simulink model "amesimcar_pathplannerv2"  (R2018b)
settings: Solver=VariableStepAuto  StartTime=0.0  StopTime=Tf  RelTol=1e-3
values from neighbouring files (symbols this model uses):
  centerline1 = line_data.centerline_right    [main.m]
  left_line = line_data.left_line    [main.m]
  right_line = line_data.right_line    [main.m]
undefined symbols (not defined in the file or in its folder): PlanningFunction
libraries: simulink x1
settings Model: Creator=pm6kgn  LastModifiedBy=t2vosx
settings DebuggingCC: LibraryContextMissingDiagnostic=none
settings SFSimCC: SimUseLocalCustomCode=off
settings RTWCC: RTWUseLocalCustomCode=off

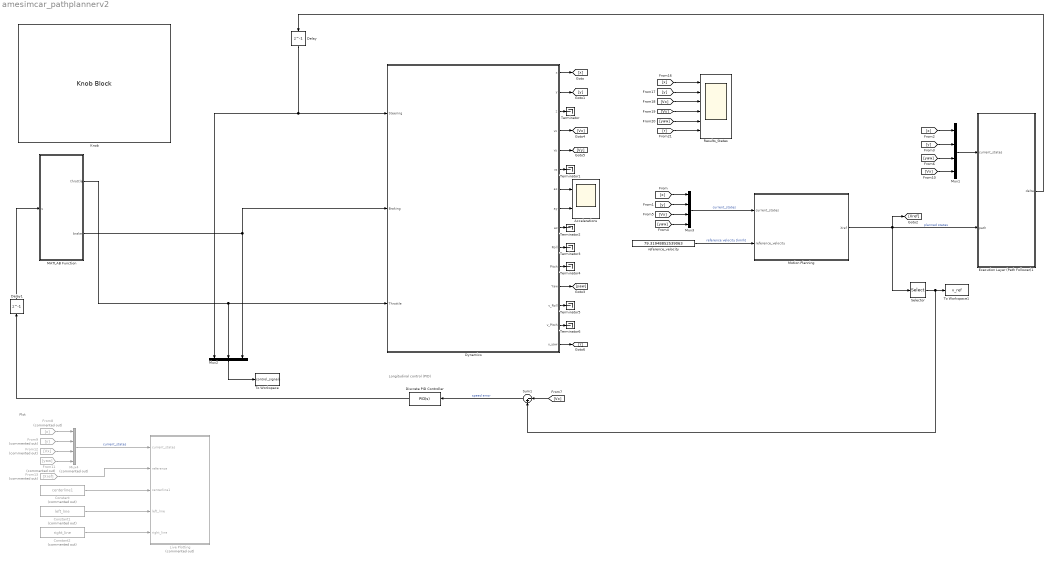
== system amesimcar_pathplannerv2 ==
  note: Plot
  note: Longitudinal control (PID)
  Accelerations : Scope  NumInputPorts=2
  Constant : Constant  Commented=on  Value=centerline1
  Constant1 : Constant  Commented=on  Value=left_line
  Constant2 : Constant  Commented=on  Value=right_line
  Delay : Delay  DelayLength=1  InitialCondition=0
  Delay1 : Delay  DelayLength=1  InitialCondition=0
  Discrete PID Controller : simulink/Continuous/PID Controller  Controller=PID  Form=Parallel  TimeDomain=Continuous-time  SampleTime=-1  IntegratorMethod=Forward Euler  FilterMethod=Forward Euler  ControllerParametersSource=internal  P=0.1  I=0.01  D=0  UseFilter=on  N=100  TunerSelectOption=Transfer Function Based (PID Tuner App)  InitialConditionSource=internal  InitialConditionForIntegrator=0  InitialConditionForFilter=0  DifferentiatorICPrevScaledInput=0  ExternalReset=none  TrackingMode=off  Kt=1  LimitOutput=on  UpperSaturationLimit=1  LowerSaturationLimit=-1  LinearizeAsGain=off  AntiWindupMode=none  Kb=1  POutMin=[]  POutMax=[]  IOutMin=[]  IOutMax=[]  DOutMin=[]  DOutMax=[]  NOutMin=[]  NOutMax=[]  SumOutMin=[]  SumOutMax=[]  SaturationOutMin=[]  SaturationOutMax=[]  PParamMin=[]  PParamMax=[]  IParamMin=[]  IParamMax=[]  DParamMin=[]  DParamMax=[]  NParamMin=[]  NParamMax=[]  KbParamMin=[]  KbParamMax=[]  KtParamMin=[]  KtParamMax=[]  KbOutMin=[]  KbOutMax=[]  KtOutMin=[]  KtOutMax=[]  IntegratorOutMin=[]  IntegratorOutMax=[]  FilterOutMin=[]  FilterOutMax=[]  SumI1OutMin=[]  SumI1OutMax=[]  SumI2OutMin=[]  SumI2OutMax=[]  SumI3OutMin=[]  SumI3OutMax=[]  SumI4OutMin=[]  SumI4OutMax=[]  SumDOutMin=[]  SumDOutMax=[]  DifferentiatorOutMin=[]  DifferentiatorOutMax=[]  FilterDiffOutCoefMin=[]  FilterDiffOutCoefMax=[]  ReciprocalOutMin=[]  ReciprocalOutMax=[]  SumDenOutMin=[]  SumDenOutMax=[]  SumNumOutMin=[]  SumNumOutMax=[]  DivideOutMin=[]  DivideOutMax=[]  IntegratorContinuousStateAttributes=''  IntegratorStateMustResolveToSignalObject=off  IntegratorRTWStateStorageClass=Auto  FilterContinuousStateAttributes=''  FilterStateMustResolveToSignalObject=off  FilterRTWStateStorageClass=Auto  ParallelPVariant=InternalParameters  IdealPVariant=Disabled  IVariant=InternalParameters  DVariant=InternalParameters  IntegratorVariant=Continuous  SatVariant=Enabled  AWVariant=Passthrough  PCopyVariant=Disabled  TRVariant=Disabled  FdbkBlocksVariant=Forward  IdealPFdbkVariant=Disabled  SatFdbkVariant=Disabled  DerivativeFilterVariant=ContFilter  NVariant=InternalParameters  NCopyVariant=Disabled  FilterICVariant=InternalICsFilter  IntegratorICVariant=InternalICs  ExternalResetVariant=Disabled  TRSumVariant=Passthrough  SumFdbkVariant=Disabled  SumVariant=Sum_PID
  Dynamics : Subsystem  Tag=AME2SLCoSim  InitFcn=AMESimLib_initBlock  StartFcn=AMESimLib_startBlock  StopFcn=AMESimLib_stopBlock
      settings: DeleteFcn=AMESimLib_deleteBlock  OpenFcn=AMESimLib_openBlock('AME2SLCoSim')
      mask Display: image(imread('amesim_pix256.png'),[0.4,0.7,0.2,0.2]);disp('Simcenter Amesim co-Sim:\nDynamics');port_label('input',1,'Steering');port_label('input',2,'Braking');port_label('input',3,'Throttle');port_label('output',1,'x');port_label('output',2,'y');port_label('output',3,'z');port_label('output',4,'vx');port_label('output',5,'vy');port_label('output',6,'vz');port_label('output',7,'ax');port_label('output',8,'ay');port_label('output',9,'az');port_label('output',10,'Roll');port_label('output',11,'Pitch');port_label('output',12,'Yaw');port_label('output',13,'v_Roll');port_label('output',14,'v_Pitch');port_label('output',15,'v_yaw');
  Execution Layer (Path Follower)1 : MATLAB Function  TreatAsAtomicUnit=on  SystemSampleTime=0.01
  From11 : From  Commented=on  GotoTag=yaw
  From12 : From  Commented=on  GotoTag=Vx
  From13 : From  Commented=on  GotoTag=Xref
  From8 : From  Commented=on  GotoTag=x
  From9 : From  Commented=on  GotoTag=y
  Knob : KnobBlock  WebBlockId=204  ScaleMin=5  ScaleMax=80
  Live Plotting : MATLAB Function  Commented=on  TreatAsAtomicUnit=on
  MATLAB Function : MATLAB Function  TreatAsAtomicUnit=on
  Motion Planning : Subsystem  TreatAsAtomicUnit=on  SystemSampleTime=0.1
      mask Display: image('C:\Users\pm6kgn\Documents\Images\2479573.png');
  Mux1 : Mux
  Mux2 : Mux  Inputs=3
  Mux3 : Mux
  Mux4 : Mux  Commented=on
  Results_States : Scope  NumInputPorts=6
  Selector : Selector  NumberOfDimensions=2  InputPortWidth=[4 50]  IndexOptions=Index vector (dialog),Index vector (dialog)  Indices=3,50  OutputSizes=1,1
  Sum1 : Sum  Inputs=|-+
  Terminator{,1..6} (7 alike) : Terminator
  To Workspace : ToWorkspace  VariableName=control_signals  SaveFormat=Structure With Time  SampleTime=-1
  To Workspace1 : ToWorkspace  VariableName=v_ref  SaveFormat=Timeseries  SampleTime=-1
  reference_velocity : Constant  Value=79.31948852539063
  wires:
  MATLAB Function/1(throttle) -> Dynamics/3(Throttle), Mux2/2
  MATLAB Function/2(brake) -> Mux2/3, Dynamics/2(Braking)
  Mux2/1 -> To Workspace/1
  Sum1/1 -> Discrete PID Controller/1  "speed error"
  Mux1/1 -> Execution Layer (Path Follower)1/1(current_states)
  Dynamics/1(x) -> [x]
  Dynamics/4(vx) -> [Vx]
  Dynamics/2(y) -> [y]
  [x] -> Mux1/1
  [y] -> Mux1/2
  Dynamics/12(Yaw) -> [yaw]
  [yaw] -> Mux1/3
  Discrete PID Controller/1 -> Delay1/1
  [Vx] -> Sum1/1
  Delay1/1 -> MATLAB Function/1(u)
  Dynamics/7(ax) -> Accelerations/1
  Dynamics/8(ay) -> Accelerations/2
  Delay/1 -> Dynamics/1(Steering), Mux2/1
  [Vx] -> Mux1/4
  Execution Layer (Path Follower)1/1(delta) -> Delay/1
  Dynamics/5(vy) -> [Vy]
  Dynamics/15(v_yaw) -> [r]
  [x] -> Results_States/1
  [y] -> Results_States/2
  [Vx] -> Results_States/3
  [Vy] -> Results_States/4
  [r] -> Results_States/6
  [yaw] -> Results_States/5
  Selector/1 -> Sum1/2, To Workspace1/1
  Motion Planning/1(Xref) -> [Xref], Selector/1, Execution Layer (Path Follower)1/2(path)  "planned states"
  [y] -> Mux3/2
  [x] -> Mux3/1
  [yaw] -> Mux3/4
  Mux3/1 -> Motion Planning/1("current_states ")  "current_states"
  [Vx] -> Mux3/3
  reference_velocity/1 -> Motion Planning/2(reference_velocity)  "reference velocity [km/h]"
  Dynamics/3(z) -> Terminator/1
  Dynamics/6(vz) -> Terminator1/1
  Dynamics/9(az) -> Terminator2/1
  Dynamics/10(Roll) -> Terminator3/1
  Dynamics/11(Pitch) -> Terminator4/1
  Dynamics/13(v_Roll) -> Terminator5/1
  Dynamics/14(v_Pitch) -> Terminator6/1
  From8/1 -> Mux4/1
  From9/1 -> Mux4/2
  Mux4/1 -> Live Plotting/1(current_states)  "current_states"
  From12/1 -> Mux4/3
  From11/1 -> Mux4/4
  From13/1 -> Live Plotting/2(reference)
  Constant/1 -> Live Plotting/3(centerline1)
  Constant1/1 -> Live Plotting/4(left_line)
  Constant2/1 -> Live Plotting/5(right_line)

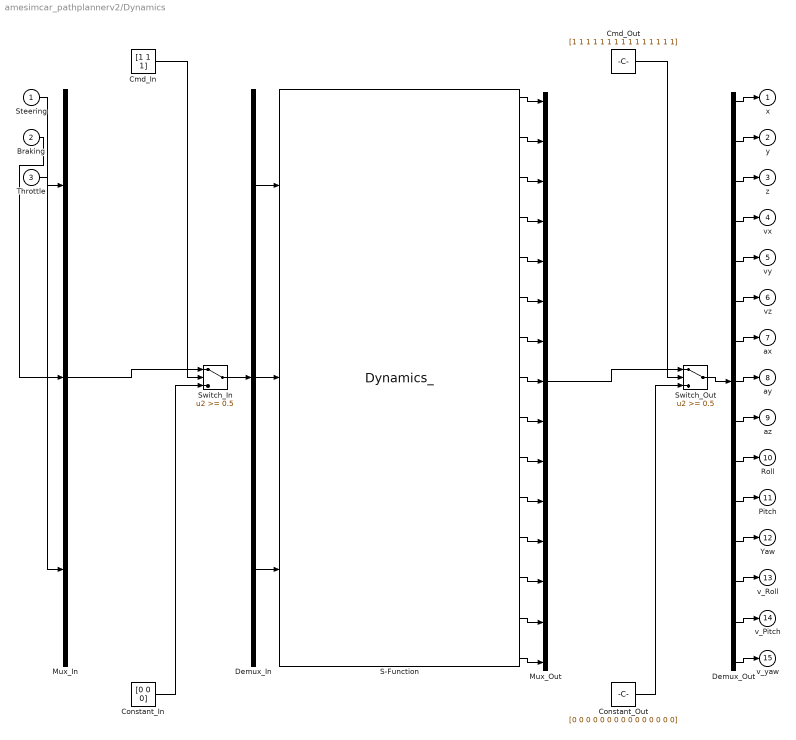
== system amesimcar_pathplannerv2/Dynamics ==
  Steering : Inport
  Braking : Inport  Port=2
  Throttle : Inport  Port=3
  Cmd_In : Constant  Value=[1 1 1]
  Cmd_Out : Constant  Value=[1 1 1 1 1 1 1 1 1 1 1 1 1 1 1]
  Constant_In : Constant  Value=[0 0 0]
  Constant_Out : Constant  Value=[0 0 0 0 0 0 0 0 0 0 0 0 0 0 0]
  Demux_In : Demux  Outputs=3
  Demux_Out : Demux  Outputs=15
  Mux_In : Mux  Inputs=3
  Mux_Out : Mux  Inputs=15
  S-Function : S-Function  InitFcn=clear Dynamics_  StopFcn=clear Dynamics_  FunctionName=Dynamics_  Parameters="[0.01;0.01;1e-05;1e+30;100;0;0;2;0;1;0.001;0;1] ['Grav           ';'Xg             ';'Zg             ';'V0             ';'Msprung        ';'Msteer         ';'Msp_front      ';'Mwh_front      ';'Msp_rear       ';'Mwh_rear       ';'Isprung_xx     ';'Isprung_yy     ';'Isprung_zz     ';'Isprung_xy     ';'Isprung_xz     ';'Isprung_yz     ';'Zref_front     ';'Zref_rear      ';'wheelbase      ';'track_front    ';'track_rear     ';'Rpinion        ';'Ksusp_front    ';'Ksusp_rear     ';'Rsusp_front    ';'Rsusp_rear     ';'Kantiroll_front';'Kantiroll_rear ';'Rfree          ';'Rroll          ';'Ktire          ';'Rtire          ';'a1             ';'a2             ';'a3             ';'a4             '] [9.8066;1056;375;0;1300;2;18;18;15;14;250;1000;1300;0;-20;0;75;75;2400;1450;1450;8;21000;21000;2000;1500;30000;20000;0.292;0.291;200000;100;-50;1200;1000;5] [] [] [] []"  SFunctionDeploymentMode=off  EnableBusSupport=off
      mask Display: port_label('output',1,'x');port_label('output',2,'y');port_label('output',3,'z');port_label('output',4,'vx');port_label('output',5,'vy');port_label('output',6,'vz');port_label('output',7,'ax');port_label('output',8,'ay');port_label('output',9,'az');port_label('output',10,'Roll');port_label('output',11,'Pitch');port_label('output',12,'Yaw');port_label('output',13,'v_Roll');port_label('output',14,'v_Pitch');port_label('output',15,'v_yaw');port_label('input',1,'Steering');port_label('input',2,'Braking');port_label('input',3,'Throttle');disp('Simcenter Amesim:\n Dynamics_')
  Switch_In : Switch  Threshold=0.5  SaturateOnIntegerOverflow=on  InputSameDT=on
  Switch_Out : Switch  Threshold=0.5  SaturateOnIntegerOverflow=on  InputSameDT=on
  x : Outport
  y : Outport  Port=2
  z : Outport  Port=3
  vx : Outport  Port=4
  vy : Outport  Port=5
  vz : Outport  Port=6
  ax : Outport  Port=7
  ay : Outport  Port=8
  az : Outport  Port=9
  Roll : Outport  Port=10
  Pitch : Outport  Port=11
  Yaw : Outport  Port=12
  v_Roll : Outport  Port=13
  v_Pitch : Outport  Port=14
  v_yaw : Outport  Port=15
  wires:
  Mux_In/1 -> Switch_In/1
  Cmd_In/1 -> Switch_In/2
  Constant_In/1 -> Switch_In/3
  Switch_In/1 -> Demux_In/1
  Mux_Out/1 -> Switch_Out/1
  Cmd_Out/1 -> Switch_Out/2
  Constant_Out/1 -> Switch_Out/3
  Switch_Out/1 -> Demux_Out/1
  Steering/1 -> Mux_In/1
  Demux_In/1 -> S-Function/1
  Braking/1 -> Mux_In/2
  Demux_In/2 -> S-Function/2
  Throttle/1 -> Mux_In/3
  Demux_In/3 -> S-Function/3
  Demux_Out/1 -> x/1
  S-Function/1 -> Mux_Out/1
  Demux_Out/2 -> y/1
  S-Function/2 -> Mux_Out/2
  Demux_Out/3 -> z/1
  S-Function/3 -> Mux_Out/3
  Demux_Out/4 -> vx/1
  S-Function/4 -> Mux_Out/4
  Demux_Out/5 -> vy/1
  S-Function/5 -> Mux_Out/5
  Demux_Out/6 -> vz/1
  S-Function/6 -> Mux_Out/6
  Demux_Out/7 -> ax/1
  S-Function/7 -> Mux_Out/7
  Demux_Out/8 -> ay/1
  S-Function/8 -> Mux_Out/8
  Demux_Out/9 -> az/1
  S-Function/9 -> Mux_Out/9
  Demux_Out/10 -> Roll/1
  S-Function/10 -> Mux_Out/10
  Demux_Out/11 -> Pitch/1
  S-Function/11 -> Mux_Out/11
  Demux_Out/12 -> Yaw/1
  S-Function/12 -> Mux_Out/12
  Demux_Out/13 -> v_Roll/1
  S-Function/13 -> Mux_Out/13
  Demux_Out/14 -> v_Pitch/1
  S-Function/14 -> Mux_Out/14
  Demux_Out/15 -> v_yaw/1
  S-Function/15 -> Mux_Out/15

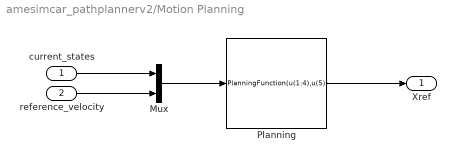
== system amesimcar_pathplannerv2/Motion Planning ==
  "current_states " : Inport
  reference_velocity : Inport  Port=2
  Mux : Mux  Inputs=2
  Planning : MATLABFcn  MATLABFcn=PlanningFunction(u(1:4),u(5))  OutputDimensions=[4,50]  Output1D=off
  Xref : Outport
  wires:
  Planning/1 -> Xref/1
  reference_velocity/1 -> Mux/2
  Mux/1 -> Planning/1
  "current_states "/1 -> Mux/1

== matlab function amesimcar_pathplannerv2/MATLAB Function ==
  data: u input; throttle output; brake output
function [throttle, brake]= fcn(u)
%#codegen

if u >= 0
    throttle = u;
    brake = 0;
else
    brake = 2*u;
    throttle = 0;
end

end

== matlab function amesimcar_pathplannerv2/Live Plotting ==
  data: current_states input; reference input; centerline1 input; left_line input; right_line input
function Plot(current_states, reference, centerline1, left_line, right_line)
    
    % Plot the reference    
    figure(1), plot(left_line(1,:), left_line(2,:), 'r', right_line(1,:), right_line(2,:), 'r', centerline1(1,:), centerline1(2,:),reference(1,:), reference(2,:),current_states(1), current_states(2), 'bo')
    
end

== matlab function amesimcar_pathplannerv2/Execution Layer (Path Follower)1 ==
  data: current_states input; delta output; path input
function delta  = PurePursuit(current_states, path)
    
    Lf = 1.056; 
    Lr = 1.344;
    L = Lf + Lr;
    G = 16.96;
    
    xCoG = current_states(1);
    yCoG = current_states(2);
    yaw = current_states(3);
    vx = current_states(4);
    
    % Pure Pursuit
    lookahead = 10;
  
    xGP = path(1,lookahead);
    yGP = path(2,lookahead);
    yawGP = path(4,lookahead);
  
    xrear = xCoG - Lr*cos(yaw);
    yrear = yCoG - Lr*sin(yaw);
    
    ld = sqrt((xGP-xrear)^2+(yGP-yrear)^2);
    
    theta_ld = atan2(yGP-yrear,xGP-xrear);
    
    alfa = -theta_ld + yaw;
    
    delta_PP = -G*atan2(2*L*sin(alfa),ld); 
    
    % Stanley Method
    
%     ks = 0.1;
%     
%     yfront = yCoG + Lf*sin(yaw);
%     xfront = xCoG + Lf*cos(yaw);
%     
%     dist_to_path = (path(1,:) - xfront).^2 + (path(2,:) - yfront).^2;            
%     [min_dist, I] = min(dist_to_path);
%                                             
%     yaw_p = path(4,I);
%     path_car_vec = [xfront-path(1,I) ; yfront-path(2,I)];
%     path_path_vec = [path(1,I) - path(1,I-1); path(2,I) - path(2,I-1)];
%     sig = det([path_car_vec, path_path_vec]);
%     deltay_p = sig*min_dist;
%     deltayaw_p = yaw - yaw_p;
%     
%     delta_S = -G*(deltayaw_p + atan2(ks*deltay_p,vx));
    
    delta = delta_PP;

end
